simulink model "myo_model_w_ctrl"  (R2020b)
settings: Solver=VariableStepAuto  StartTime=0.0  StopTime=4  RelTol=1e-3
undefined symbols (not defined in the file or in its folder): beta_force, beta_force_int, beta_pos, Kd, Kp
libraries: cstblocks x24
settings Model: Creator=simon  LastModifiedBy=nicol
settings SolverCC: ZeroCrossAlgorithm=Adaptive
settings DebuggingCC: IgnoredZcDiagnostic=none

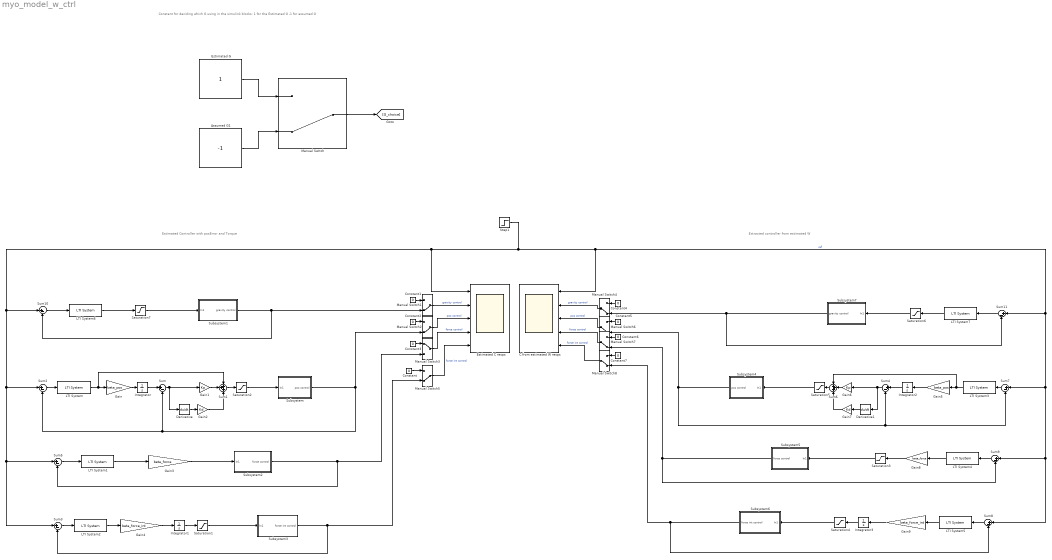
== system myo_model_w_ctrl ==
  note: Constant for deciding which G using in the simulink blocks:
      | 1 for the Estimated G
      | -1 for assumed G
  note: Estimated Controller with posError and Torque
  note: Extracted controller from estimated W
  Assumed G1 : Constant  Value=-1
  C from estimated W resps : Scope  NumInputPorts=5
  Constant{,1..7} (8 alike) : Constant  Value=0
  Derivative : Derivative
  Derivative1 : Derivative
  Estimated C resps : Scope  NumInputPorts=5
  Estimated G : Constant
  Gain : Gain  Gain=beta_pos
  Gain1 : Gain  Gain=Kp
  Gain2 : Gain  Gain=Kd
  Gain3 : Gain  Gain=beta_force
  Gain4 : Gain  Gain=beta_force_int
  Gain5 : Gain  Gain=beta_pos
  Gain6 : Gain  Gain=Kp
  Gain7 : Gain  Gain=Kd
  Gain8 : Gain  Gain=beta_force
  Gain9 : Gain  Gain=beta_force_int
  Integrator{,1..3} (4 alike) : Integrator
  LTI System{,1..2,6} (4 alike) : cstblocks/LTI System  sys=C_best  IC=[]
  LTI System{3..5,7} (4 alike) : cstblocks/LTI System  sys=C_from_Wbest  IC=[]
  Manual Switch{,1..2,4..8} (8 alike) : ManualSwitch  CurrentSetting=0
  Manual Switch3 : ManualSwitch
  Saturation{1..7} (7 alike) : Saturate  UpperLimit=6  LowerLimit=-6
  Step1 : Step  Time=0  SampleTime=0
  Subsystem : Subsystem
  Subsystem1 : Subsystem
  Subsystem2 : Subsystem
  Subsystem3 : Subsystem
  Subsystem4 : Subsystem
  Subsystem5 : Subsystem
  Subsystem6 : Subsystem
  Subsystem7 : Subsystem
  Sum{,2..5,7..11} (10 alike) : Sum  Inputs=|+-
  Sum1 : Sum  Inputs=+++
  Sum6 : Sum  Inputs=+++
  wires:
  Gain/1 -> Integrator/1
  Derivative/1 -> Gain2/1
  Sum/1 -> Derivative/1, Gain1/1
  Gain1/1 -> Sum1/2
  Gain2/1 -> Sum1/3
  Sum1/1 -> Saturation2/1
  Integrator/1 -> Sum/1
  LTI System/1 -> Sum1/1, Gain/1
  Sum2/1 -> LTI System/1
  Sum5/1 -> LTI System1/1
  LTI System2/1 -> Gain4/1
  Gain4/1 -> Integrator1/1
  Sum3/1 -> LTI System2/1
  Integrator1/1 -> Saturation1/1
  Sum9/1 -> LTI System4/1
  Integrator3/1 -> Saturation4/1
  LTI System3/1 -> Gain5/1, Sum6/1
  Sum7/1 -> LTI System3/1
  LTI System5/1 -> Gain9/1
  LTI System4/1 -> Gain8/1
  Gain9/1 -> Integrator3/1
  Gain8/1 -> Saturation3/1
  Sum8/1 -> LTI System5/1
  Integrator2/1 -> Sum4/1
  Derivative1/1 -> Gain7/1
  Sum6/1 -> Saturation5/1
  Sum4/1 -> Derivative1/1, Gain6/1
  Gain6/1 -> Sum6/2
  Gain7/1 -> Sum6/3
  Gain5/1 -> Integrator2/1
  LTI System1/1 -> Gain3/1
  LTI System6/1 -> Saturation7/1
  Sum10/1 -> LTI System6/1
  Step1/1 -> Sum8/1, Sum9/1, Sum7/1, Sum11/1, C from estimated W resps/1, Sum3/1, Sum5/1, Sum2/1, Sum10/1, Estimated C resps/1  "ref"
  Sum11/1 -> LTI System7/1
  LTI System7/1 -> Saturation6/1
  Manual Switch1/1 -> Estimated C resps/2  "gravity control"
  Manual Switch2/1 -> Estimated C resps/3  "pos control"
  Manual Switch3/1 -> Estimated C resps/4  "force control"
  Manual Switch5/1 -> Estimated C resps/5  "force int control"
  Manual Switch4/1 -> C from estimated W resps/2  "gravity control"
  Manual Switch7/1 -> C from estimated W resps/4  "force control"
  Manual Switch6/1 -> C from estimated W resps/3  "pos control"
  Manual Switch8/1 -> C from estimated W resps/5  "force int control"
  Manual Switch/1 -> [G_choice]
  Estimated G/1 -> Manual Switch/1
  Assumed G1/1 -> Manual Switch/2
  Constant/1 -> Manual Switch5/1
  Constant1/1 -> Manual Switch1/1
  Constant2/1 -> Manual Switch2/1
  Constant3/1 -> Manual Switch3/1
  Constant4/1 -> Manual Switch4/1
  Constant5/1 -> Manual Switch6/1
  Constant6/1 -> Manual Switch7/1
  Constant7/1 -> Manual Switch8/1
  Subsystem/1(pos control) -> Manual Switch2/2, Sum/2, Sum2/2
  Saturation2/1 -> Subsystem/1(In1)
  Subsystem1/1(gravity control) -> Manual Switch1/2, Sum10/2
  Saturation7/1 -> Subsystem1/1(In1)
  Subsystem2/1(force control) -> Manual Switch3/2, Sum5/2
  Gain3/1 -> Subsystem2/1(In1)
  Subsystem3/1(force int control) -> Manual Switch5/2, Sum3/2
  Saturation1/1 -> Subsystem3/1(In1)
  Subsystem4/1(pos control) -> Sum7/2, Sum4/2, Manual Switch6/2
  Saturation5/1 -> Subsystem4/1(In1)
  Subsystem5/1(force control) -> Manual Switch7/2, Sum9/2
  Saturation3/1 -> Subsystem5/1(In1)
  Subsystem6/1(force int control) -> Sum8/2, Manual Switch8/2
  Saturation4/1 -> Subsystem6/1(In1)
  Subsystem7/1(gravity control) -> Sum11/2, Manual Switch4/2
  Saturation6/1 -> Subsystem7/1(In1)

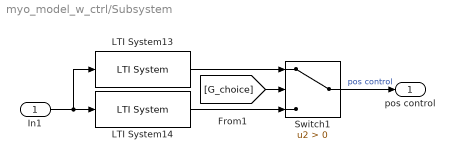
== system myo_model_w_ctrl/Subsystem ==
  In1 : Inport
  LTI System13 : cstblocks/LTI System  sys=G_best  IC=[]
  LTI System14 : cstblocks/LTI System  sys=G_assumed  IC=[]
  Switch1 : Switch  Criteria=u2 > Threshold
  pos control : Outport
  wires:
  In1/1 -> LTI System13/1, LTI System14/1
  LTI System13/1 -> Switch1/1
  Switch1/1 -> pos control/1  "pos control"
  LTI System14/1 -> Switch1/3
  [G_choice] -> Switch1/2

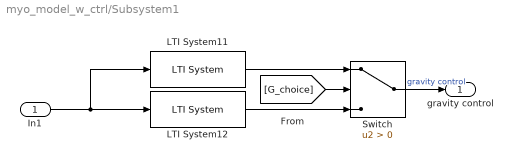
== system myo_model_w_ctrl/Subsystem1 ==
  In1 : Inport
  LTI System11 : cstblocks/LTI System  sys=G_best  IC=[]
  LTI System12 : cstblocks/LTI System  sys=G_assumed  IC=[]
  Switch : Switch  Criteria=u2 > Threshold
  gravity control : Outport
  wires:
  LTI System12/1 -> Switch/3
  Switch/1 -> gravity control/1  "gravity control"
  In1/1 -> LTI System12/1, LTI System11/1
  [G_choice] -> Switch/2
  LTI System11/1 -> Switch/1

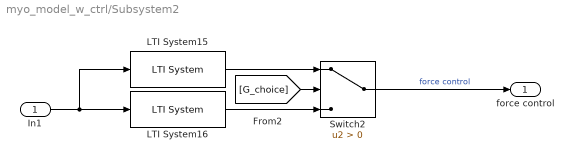
== system myo_model_w_ctrl/Subsystem2 ==
  In1 : Inport
  LTI System15 : cstblocks/LTI System  sys=G_best  IC=[]
  LTI System16 : cstblocks/LTI System  sys=G_assumed  IC=[]
  Switch2 : Switch  Criteria=u2 > Threshold
  force control : Outport
  wires:
  [G_choice] -> Switch2/2
  LTI System15/1 -> Switch2/1
  LTI System16/1 -> Switch2/3
  Switch2/1 -> force control/1  "force control"
  In1/1 -> LTI System15/1, LTI System16/1

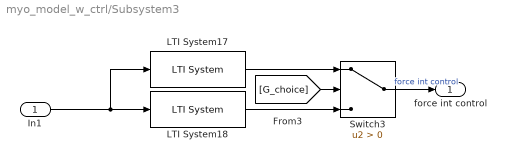
== system myo_model_w_ctrl/Subsystem3 ==
  In1 : Inport
  LTI System17 : cstblocks/LTI System  sys=G_best  IC=[]
  LTI System18 : cstblocks/LTI System  sys=G_assumed  IC=[]
  Switch3 : Switch  Criteria=u2 > Threshold
  force int control : Outport
  wires:
  LTI System18/1 -> Switch3/3
  In1/1 -> LTI System17/1, LTI System18/1
  [G_choice] -> Switch3/2
  LTI System17/1 -> Switch3/1
  Switch3/1 -> force int control/1  "force int control"

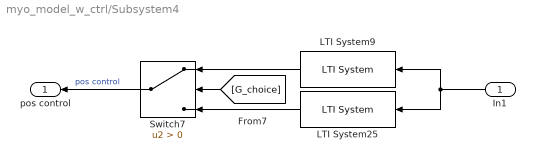
== system myo_model_w_ctrl/Subsystem4 ==
  In1 : Inport
  LTI System25 : cstblocks/LTI System  sys=G_assumed  IC=[]
  LTI System9 : cstblocks/LTI System  sys=G_best  IC=[]
  Switch7 : Switch  Criteria=u2 > Threshold
  pos control : Outport
  wires:
  [G_choice] -> Switch7/2
  LTI System25/1 -> Switch7/3
  In1/1 -> LTI System9/1, LTI System25/1
  Switch7/1 -> pos control/1  "pos control"
  LTI System9/1 -> Switch7/1

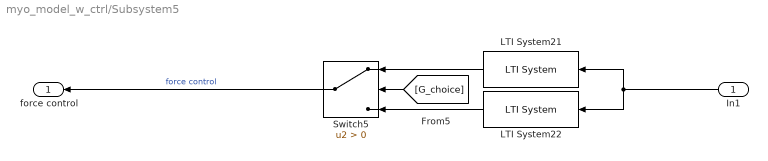
== system myo_model_w_ctrl/Subsystem5 ==
  In1 : Inport
  LTI System21 : cstblocks/LTI System  sys=G_best  IC=[]
  LTI System22 : cstblocks/LTI System  sys=G_assumed  IC=[]
  Switch5 : Switch  Criteria=u2 > Threshold
  force control : Outport
  wires:
  In1/1 -> LTI System22/1, LTI System21/1
  LTI System22/1 -> Switch5/3
  Switch5/1 -> force control/1  "force control"
  [G_choice] -> Switch5/2
  LTI System21/1 -> Switch5/1

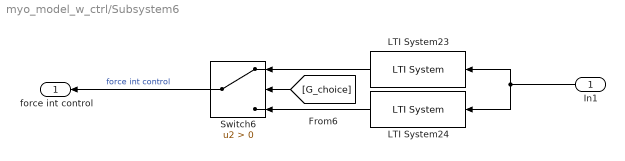
== system myo_model_w_ctrl/Subsystem6 ==
  In1 : Inport
  LTI System23 : cstblocks/LTI System  sys=G_best  IC=[]
  LTI System24 : cstblocks/LTI System  sys=G_assumed  IC=[]
  Switch6 : Switch  Criteria=u2 > Threshold
  force int control : Outport
  wires:
  In1/1 -> LTI System24/1, LTI System23/1
  [G_choice] -> Switch6/2
  LTI System23/1 -> Switch6/1
  LTI System24/1 -> Switch6/3
  Switch6/1 -> force int control/1  "force int control"

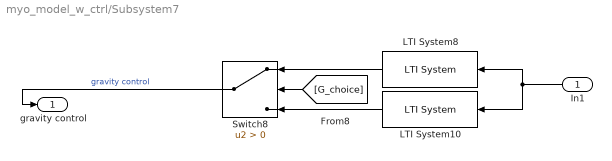
== system myo_model_w_ctrl/Subsystem7 ==
  In1 : Inport
  LTI System10 : cstblocks/LTI System  sys=G_assumed  IC=[]
  LTI System8 : cstblocks/LTI System  sys=G_best  IC=[]
  Switch8 : Switch  Criteria=u2 > Threshold
  gravity control : Outport
  wires:
  In1/1 -> LTI System10/1, LTI System8/1
  LTI System10/1 -> Switch8/3
  Switch8/1 -> gravity control/1  "gravity control"
  [G_choice] -> Switch8/2
  LTI System8/1 -> Switch8/1
